simulink model "sensorless"  (R2018b)
settings: Solver=ode45  StartTime=0.0  StopTime=0.5  RelTol=1e-3  EnableMultiTasking=on
InitFcn:
  | tpwm=0.0001;
  | K=0.0604;
  | L1=0.00248;
  | L2=-1.239e-7*40;
  | Td=0;
  | kr=50;
  | wc=5;
  | speedref=10;
  | L1=0.00248;
  | L2=-1.239e-7*200;
libraries: dspsigops x72, powerlib x31, powerlib_meascontrol x24, simulink x8, powerlib_extras x5
(part 1 of 2)
settings Model: SimulationMode=accelerator  Creator=Administrator  LastModifiedBy=chenhao
settings DataIOCC: LimitDataPoints=on  SaveFormat=Array
settings OptimizationCC: EfficientMapNaN2IntZero=off  LifeSpan=inf
settings DebuggingCC: UnderspecifiedInitializationDetection=Classic  MergeDetectMultiDrivingBlocksExec=none  SolverPrmCheckMsg=warning  AllowSymbolicDim=off  SFUnexpectedBacktrackingDiag=warning  SFNoUnconditionalDefaultTransitionDiag=warning  SFExecutionAtInitializationDiag=none
settings HardwareCC: ProdBitPerPointer=32  ProdBitPerSizeT=32  ProdBitPerPtrDiffT=32  ProdLargestAtomicFloat=None  ProdIntDivRoundTo=Undefined  ProdEndianess=Unspecified  ProdWordSize=32  ProdHWDeviceType=32-bit Generic  TargetBitPerPointer=64  TargetBitPerSizeT=64  TargetBitPerPtrDiffT=64  TargetLongLongMode=on  TargetIntDivRoundTo=Zero  TargetEndianess=LittleEndian  TargetWordSize=64  TargetHWDeviceType=MATLAB Host  ProdEqTarget=off
settings ModelReferenceCC: PropagateSignalLabelsOutOfModel=off
settings SFSimCC: SimUseLocalCustomCode=off
settings RTWCC: RTWUseLocalCustomCode=off
settings CodeAppCC: MaxIdLength=128  StateflowObjectComments=on
settings GRTTargetCC: TargetLangStandard=C89/C90 (ANSI)  CombineOutputUpdateFcns=off  GRTInterface=on
settings ConfigComp: CovMetricSettings=dw  CovHtmlReporting=on  CovSaveCumulativeToWorkspaceVar=on  CovSaveSingleToWorkspaceVar=on  CovExternalEMLEnable=off
settings SimscapeCC: SimscapeNormalizeSystem=off

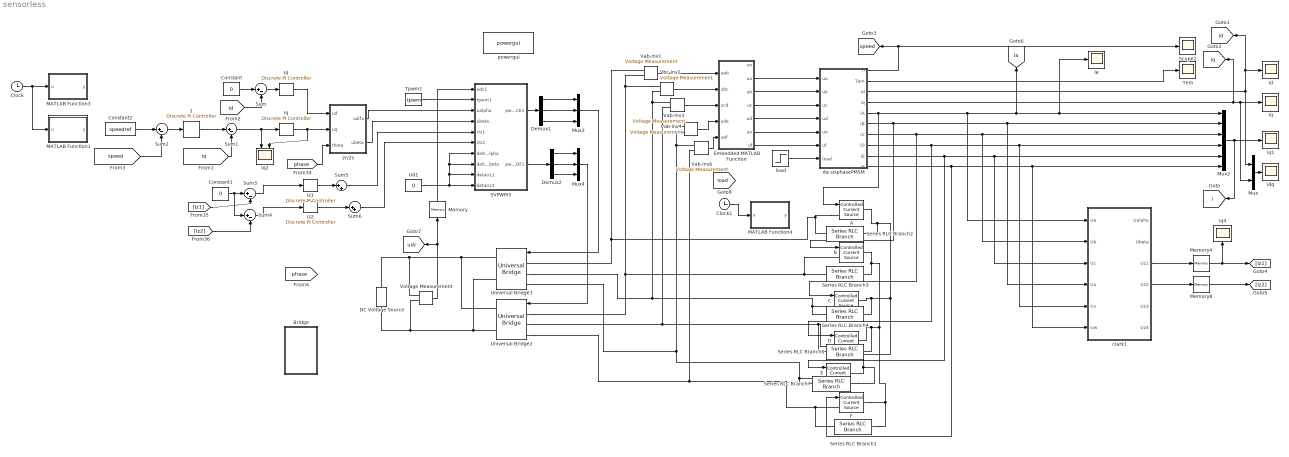
== system sensorless ==
  "    1" : powerlib_extras/Discrete  Control Blocks/Discrete PI Controller  Kp=1  Ki=80  Par_Limits=[50 -50]  Init=0  Ts=tpwm
  " Id" : powerlib_extras/Discrete  Control Blocks/Discrete PI Controller  Kp=3  Ki=120  Par_Limits=[300 -300]  Init=0  Ts=tpwm
  " Iq" : powerlib_extras/Discrete  Control Blocks/Discrete PI Controller  Kp=3  Ki=120  Par_Limits=[300 -300]  Init=0  Ts=tpwm
  " iz1" : powerlib_extras/Discrete  Control Blocks/Discrete PI Controller  Kp=10  Ki=100  Par_Limits=[300 -300]  Init=0  Ts=tpwm
  " iz2" : powerlib_extras/Discrete  Control Blocks/Discrete PI Controller  Kp=10  Ki=100  Par_Limits=[300 -300]  Init=0  Ts=tpwm
  2r/2s : Subsystem
  A : powerlib/Electrical Sources/Controlled Current Source  Initialize=on  Source_Type=AC  Amplitude=0  Phase=0  Frequency=0  Measurements=None
  B : powerlib/Electrical Sources/Controlled Current Source  Initialize=on  Source_Type=AC  Amplitude=0  Phase=0  Frequency=0  Measurements=None
  Bridge : Subsystem
  C : powerlib/Electrical Sources/Controlled Current Source  Initialize=on  Source_Type=AC  Amplitude=0  Phase=0  Frequency=0  Measurements=None
  Clock : Clock
  Clock1 : Clock
  Constant : Constant  Value=0
  Constant1 : Constant  Value=0
  Constant2 : Constant  Value=speedref
  D : powerlib/Electrical Sources/Controlled Current Source  Initialize=on  Source_Type=AC  Amplitude=0  Phase=0  Frequency=0  Measurements=None
  DC Voltage Source : powerlib/Electrical Sources/DC Voltage Source  Amplitude=100  Measurements=Voltage
  Demux1 : Demux  Outputs=3
  Demux2 : Demux  Outputs=3
  E : powerlib/Electrical Sources/Controlled Current Source  Initialize=on  Source_Type=AC  Amplitude=0  Phase=0  Frequency=0  Measurements=None
  Embedded MATLAB Function : MATLAB Function  TreatAsAtomicUnit=on
  F : powerlib/Electrical Sources/Controlled Current Source  Initialize=on  Source_Type=AC  Amplitude=0  Phase=0  Frequency=0  Measurements=None
  Ia : Scope
  MATLAB Function1 : MATLAB Function  TreatAsAtomicUnit=on
  MATLAB Function3 : MATLAB Function  TreatAsAtomicUnit=on
  MATLAB Function4 : MATLAB Function  TreatAsAtomicUnit=on
  Memory : Memory
  Memory4 : Memory
  Memory8 : Memory
  Mux : Mux  Inputs=2
  Mux2 : Mux  Inputs=6
  Mux3 : Mux  Inputs=3
  Mux4 : Mux  Inputs=3
  SVPWM3 : Subsystem
  Scope2 : Scope
  Series RLC Branch{1..4,6..7} (6 alike) : powerlib/Elements/Series RLC Branch  LConnTagsString=__new0  RConnTagsString=__new0  BranchType=R  Resistance=10e10  Inductance=10e-7  SetiL0=off  InitialCurrent=0  Capacitance=1e-6  Setx0=off  InitialVoltage=0  Measurements=None
  Sum{,1..4} (5 alike) : Sum  Inputs=|+-
  Sum5 : Sum  Inputs=|++
  Sum6 : Sum  Inputs=|++
  Tem : Scope
  Tpwm1 : Constant  Value=tpwm
  Ud1 : Constant  Value=0
  Universal Bridge1 : powerlib/Power Electronics/Universal Bridge  Arms=3  SnubberResistance=1e5  SnubberCapacitance=inf  Device=IGBT / Diodes  Ron=1e-3  Lon=0  ForwardVoltages="[  0  0  ]"  ForwardVoltage=0  GTOparameters=[ 10e-6 , 20e-6 ]  IGBTparameters=[ 0 , 0 ]  Measurements=None  Measurements_2=None  converterType=Rectifier
  Universal Bridge2 : powerlib/Power Electronics/Universal Bridge  Arms=3  SnubberResistance=1e5  SnubberCapacitance=inf  Device=IGBT / Diodes  Ron=1e-3  Lon=0  ForwardVoltages="[  0  0  ]"  ForwardVoltage=0  GTOparameters=[ 10e-6 , 20e-6 ]  IGBTparameters=[ 0 , 0 ]  Measurements=None  Measurements_2=None  converterType=Rectifier
  Vab-inv{1,3..4,6} (4 alike) : powerlib/Measurements/Voltage Measurement  Tag=PoWeRsYsTeMmEaSuReMeNt  PhasorSimulation=off  OutputType=Magnitude  PSBequivalent=0
  Vbc-inv2 : powerlib/Measurements/Voltage Measurement  Tag=PoWeRsYsTeMmEaSuReMeNt  PhasorSimulation=off  OutputType=Magnitude  PSBequivalent=0
  Voltage Measurement : powerlib/Measurements/Voltage Measurement  PhasorSimulation=off  OutputType=Complex  PSBequivalent=0
  clark1 : MATLAB Function  TreatAsAtomicUnit=on
  dq-sixphasePMSM : Subsystem  mask{R=0.099, Ld=2.463342136542000e-03, Lq=2.473254136542000e-03, Lf=1.520747e-3, psi=0.0592, p=5, J=0.00174}
      mask prompts: R "Resistance (Om)"; Ld "d-inductance (H)"; Lq "q-inductance (H)"; Lf "Leak inductance (H)"; psi "flux (Wb)"; p "pole pairs"; J "inertia (kg*m^2)"
  id : Scope
  idq : Scope
  iq : Scope
  iq1 : Scope
  iq2 : Scope  NumInputPorts=2
  iq4 : Scope
  load : Step  Time=0.1  After=5  SampleTime=0
  powergui : powerlib/powergui  Priority=1  SimulationMode=Discrete  SampleTime=5e-7  frequency=60  Iterations=50  frequencyindice=0  Pbase=100e6  ErrMax=1e-4  UnitsV=kV  UnitsW=MW  buscounter=0  FunctionMessages=off  echomessages=off  EnableUseOfTLC=off  CurrentSourceSwitches=off  DisableSnubberDevices=off  DisableRonSwitches=off  DisableVfSwitches=off  DisplayEquations=off  SolverType=Tustin  Interpol=off  ExternalGateDelay=off  methode=off  Ts=0  x0status=blocks  SPID=off  SwTol=0  HookPort=off  RestoreLinks=warning  ResistiveCurrentMeasurement=off  Frange=[0:2:500]  Ylog=off  Xlog=on  ShowGrid=off  save=off  variable=ZData  structure=Ia  ZoomFFT=on  StartTime=0.1  cycles=2  DisplayStyle=1  fundamental=2.5  FreqAxis=on  MaxFrequency=30  frequencyindicesteady=1  RmsSteady=1  display=off
  tag scope: Ia=global, i=global, id=global, iq=global, load=global, speed=global, udc=global
  wires:
  Vab-inv1/1 -> Embedded MATLAB Function/1(uab)
  Vbc-inv2/1 -> Embedded MATLAB Function/2(ubc)
  Vab-inv3/1 -> Embedded MATLAB Function/3(ucd)
  Vab-inv4/1 -> Embedded MATLAB Function/4(ude)
  Vab-inv6/1 -> Embedded MATLAB Function/5(uef)
  Embedded MATLAB Function/2(ua) -> dq-sixphasePMSM/1(ua)
  Embedded MATLAB Function/3(ub) -> dq-sixphasePMSM/2(ub)
  Embedded MATLAB Function/4(uc) -> dq-sixphasePMSM/3(uc)
  Embedded MATLAB Function/5(ud) -> dq-sixphasePMSM/4(ud)
  Embedded MATLAB Function/6(ue) -> dq-sixphasePMSM/5(ue)
  Embedded MATLAB Function/7(uf) -> dq-sixphasePMSM/6(uf)
  Mux/1 -> idq/1
  Sum1/1 -> iq2/1, " Iq"/1
  Constant/1 -> Sum/1
  Sum2/1 -> "    1"/1
  [phase] -> 2r/2s/3(theta)
  Mux3/1 -> Universal Bridge1/1
  Demux1/2 -> Mux3/2
  Mux4/1 -> Universal Bridge2/1
  Mux2/1 -> iq1/1, [i]
  "    1"/1 -> Sum1/1
  Sum/1 -> " Id"/1
  " Id"/1 -> 2r/2s/1(ud)
  " Iq"/1 -> iq2/2, 2r/2s/2(uq)
  Demux2/2 -> Mux4/2
  Demux2/1 -> Mux4/1
  Demux1/3 -> Mux3/3
  Demux2/3 -> Mux4/3
  Voltage Measurement/1 -> [udc], Memory/1
  SVPWM3/1(pwm_ACE1) -> Demux1/1
  SVPWM3/2(pwm_BDF1) -> Demux2/1
  dq-sixphasePMSM/1(n) -> Scope2/1, [speed]
  dq-sixphasePMSM/2(Tem) -> Tem/1
  dq-sixphasePMSM/3(id) -> [id], id/1, Mux/1
  dq-sixphasePMSM/4(iq) -> [iq], Mux/2, iq/1
  dq-sixphasePMSM/5(iA) -> A/1, clark1/1(Ua), [Ia], Ia/1, Mux2/1
  dq-sixphasePMSM/6(iB) -> B/1, clark1/4(Uu), Mux2/2
  dq-sixphasePMSM/7(iC) -> C/1, clark1/2(Ub), Mux2/3
  dq-sixphasePMSM/8(iD) -> D/1, clark1/5(Uv), Mux2/4
  dq-sixphasePMSM/10(iF) -> F/1, clark1/6(Uw), Mux2/6
  dq-sixphasePMSM/9(iE) -> E/1, clark1/3(Uc), Mux2/5
  [id] -> Sum/2
  [iq] -> Sum1/2
  Tpwm1/1 -> SVPWM3/2(tpwm1)
  Memory/1 -> SVPWM3/1(udc1)
  2r/2s/1(ualfa) -> SVPWM3/3(ualpha)
  2r/2s/2(ubeta) -> SVPWM3/4(ubeta)
  Constant1/1 -> Sum4/1, Sum3/1
  Sum3/1 -> " iz1"/1
  Sum4/1 -> " iz2"/1
  Ud1/1 -> SVPWM3/9(detaUz1), SVPWM3/8(deltaUbeta), SVPWM3/7(deltaUalpha), SVPWM3/10(detaUz2)
  " iz1"/1 -> Sum5/1
  " iz2"/1 -> Sum6/1
  clark1/3(Uz1) -> Memory4/1
  clark1/4(Uz2) -> Memory8/1
  Memory4/1 -> [Iz1], iq4/1
  Memory8/1 -> [Iz2]
  [Iz1] -> Sum3/2
  [Iz2] -> Sum4/2
  Demux1/1 -> Mux3/1
  Clock/1 -> MATLAB Function1/1(u), MATLAB Function3/1(u)
  Clock1/1 -> MATLAB Function4/1(u)
  [speed] -> Sum2/2
  Sum5/1 -> SVPWM3/5(Uz1)
  Sum6/1 -> SVPWM3/6(Uz2)
  load/1 -> dq-sixphasePMSM/7(load)
  Constant2/1 -> Sum2/1
  connections:
  A/LConn1 -- Series RLC Branch2/LConn1 -- Universal Bridge1/LConn1 -- Vab-inv1/LConn1
  Vbc-inv2/LConn1 -- Universal Bridge2/LConn1 -- Series RLC Branch3/LConn1 -- B/LConn1 -- Vab-inv1/LConn2
  C/LConn1 -- Universal Bridge1/LConn2 -- Vbc-inv2/LConn2 -- Vab-inv3/LConn1 -- Series RLC Branch4/LConn1
  Vab-inv4/LConn1 -- Vab-inv3/LConn2 -- Series RLC Branch6/LConn1 -- D/LConn1 -- Universal Bridge2/LConn2
  E/LConn1 -- Universal Bridge1/LConn3 -- Vab-inv4/LConn2 -- Vab-inv6/LConn1 -- Series RLC Branch7/LConn1
  Series RLC Branch1/LConn1 -- F/LConn1 -- Universal Bridge2/LConn3 -- Vab-inv6/LConn2
  Series RLC Branch1/RConn1 -- F/RConn1 -- Series RLC Branch3/RConn1 -- B/RConn1 -- Series RLC Branch6/RConn1 -- D/RConn1
  Series RLC Branch7/RConn1 -- E/RConn1 -- Series RLC Branch2/RConn1 -- A/RConn1 -- Series RLC Branch4/RConn1 -- C/RConn1
  Universal Bridge2/RConn2 -- DC Voltage Source/LConn1 -- Voltage Measurement/LConn2 -- Universal Bridge1/RConn2
  Universal Bridge2/RConn1 -- Universal Bridge1/RConn1 -- DC Voltage Source/RConn1 -- Voltage Measurement/LConn1

== system sensorless/2r//2s ==
  ud : Inport
  uq : Inport  Port=2
  theta : Inport  Port=3
  Fcn : Fcn  Expr=u(1)*cos(u(3))-u(2)*sin(u(3))
  Fcn1 : Fcn  Expr=u(1)*sin(u(3))+u(2)*cos(u(3))
  Mux1 : Mux  Inputs=3
  ualfa : Outport
  ubeta : Outport  Port=2
  wires:
  theta/1 -> Mux1/3
  uq/1 -> Mux1/2
  ud/1 -> Mux1/1
  Fcn1/1 -> ubeta/1
  Fcn/1 -> ualfa/1
  Mux1/1 -> Fcn1/1, Fcn/1

== system sensorless/Bridge ==
  100uF : powerlib/Elements/Series RLC Branch  LConnTagsString=__new0  RConnTagsString=__new0  BranchType=C  Resistance=1  Inductance=1e-3  SetiL0=off  InitialCurrent=0  Capacitance=1000e-6  Setx0=on  InitialVoltage=500  Measurements=None
  Diode{,1..5} (6 alike) : powerlib/Power Electronics/Diode  Ron=0.001  Lon=0  Vf=0.8  IC=0  UseSnubber=off  Rs=500  Cs=250e-9  Measurements=on
  Three-Phase Source1 : powerlib/Electrical Sources/Three-Phase Source  InternalConnection=Yg  VoltagePhases=off  Voltage=380  PhaseAngle=0  Voltage_phases=[25e3 25e3 25e3]/sqrt(3)  PhaseAngles_phases=[0 -120 +120]  Frequency=50  NonIdealSource=on  SpecifyImpedance=off  Resistance=1  Inductance=0.0000075  ShortCircuitLevel=100e6  BaseVoltage=380  XRratio=7  BusType=swing  Pref=0  Qref=0  Prefabc=[10e3, 10e3, 10e3]  Qrefabc=[0, 0, 0]  Qmin=-inf  Qmax=inf
  filter : powerlib/Elements/Series RLC Branch  LConnTagsString=__new0  RConnTagsString=__new0  BranchType=L  Resistance=1  Inductance=1e-6  SetiL0=off  InitialCurrent=0  Capacitance=1e-6  Setx0=off  InitialVoltage=0  Measurements=None
  +Vdc : PMIOPort  Tag=PMCPort  Side=Left
  -Vdc : PMIOPort  Tag=PMCPort  Port=2  Side=Right
  connections:
  filter/LConn1 -- Diode1/RConn1 -- Diode/RConn1 -- Diode4/RConn1
  Diode3/LConn1 -- Diode5/LConn1 -- Diode2/LConn1 -- 100uF/RConn1 -- -Vdc/RConn1
  Three-Phase Source1/RConn1 -- Diode2/RConn1 -- Diode/LConn1
  Diode3/RConn1 -- Three-Phase Source1/RConn3 -- Diode4/LConn1
  Three-Phase Source1/RConn2 -- Diode5/RConn1 -- Diode1/LConn1
  100uF/LConn1 -- +Vdc/RConn1 -- filter/RConn1

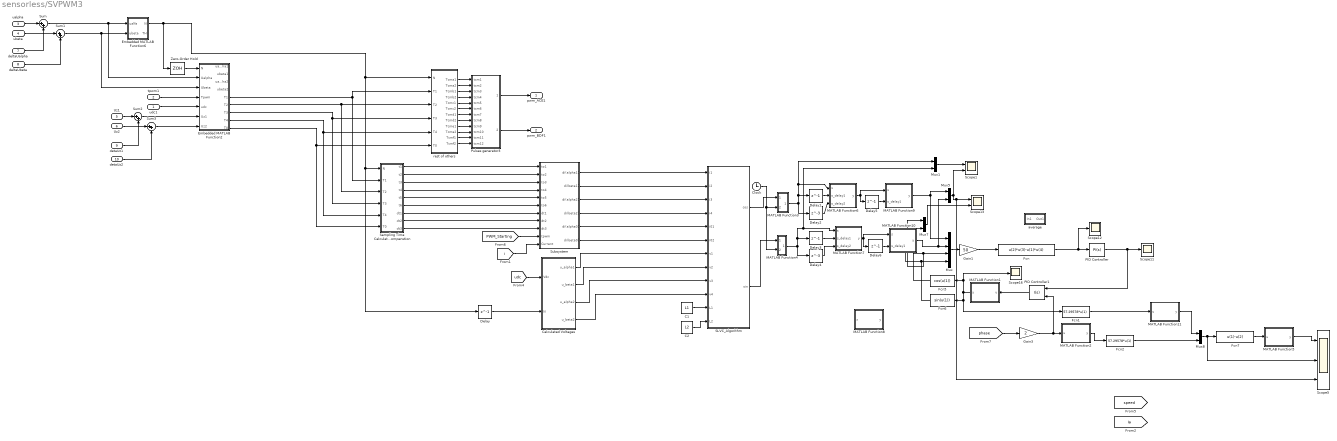
== system sensorless/SVPWM3 ==
  udc1 : Inport
  tpwm1 : Inport  Port=2
  ualpha : Inport  Port=3
  ubeta : Inport  Port=4
  Uz1 : Inport  Port=5
  Uz2 : Inport  Port=6
  deltaUalpha : Inport  Port=7
  deltaUbeta : Inport  Port=8
  detaUz1 : Inport  Port=9
  detaUz2 : Inport  Port=10
  C1 : Constant  Value=L1
  C2 : Constant  Value=L2
  "Calculated Voltages " : Subsystem
  Clock : Clock
  Delay{,1,3,5..6} (5 alike) : Delay  DelayLength=1  InitialCondition=0  SampleTime=1e-4
  Delay2 : Delay  DelayLength=3  InitialCondition=0  SampleTime=1e-4
  Delay4 : Delay  DelayLength=3  InitialCondition=0  SampleTime=1e-4
  Embedded MATLAB Function2 : MATLAB Function  TreatAsAtomicUnit=on
  Embedded MATLAB Function6 : MATLAB Function  TreatAsAtomicUnit=on
  Fcn : Fcn  Expr=u(2)*u(3)-u(1)*u(4)
  Fcn1 : Fcn  Expr=57.29578*u(1)
  Fcn2 : Fcn  Expr=57.29578*u(1)
  Fcn5 : Fcn  Expr=cos(u(1))
  Fcn6 : Fcn  Expr=sin(u(1))
  Fcn7 : Fcn  Expr=u(1)-u(2)
  Gain1 : Gain  Gain=50
  Gain3 : Gain  Gain=2
  MATLAB Function1 : MATLAB Function  TreatAsAtomicUnit=on
  MATLAB Function10 : MATLAB Function  TreatAsAtomicUnit=on
  MATLAB Function11 : MATLAB Function  TreatAsAtomicUnit=on
  MATLAB Function2 : MATLAB Function  TreatAsAtomicUnit=on
  MATLAB Function3 : MATLAB Function  TreatAsAtomicUnit=on
  MATLAB Function4 : MATLAB Function  TreatAsAtomicUnit=on
  MATLAB Function5 : MATLAB Function  TreatAsAtomicUnit=on
  MATLAB Function6 : MATLAB Function  TreatAsAtomicUnit=on
  MATLAB Function7 : MATLAB Function  TreatAsAtomicUnit=on
  MATLAB Function8 : MATLAB Function  TreatAsAtomicUnit=on
  MATLAB Function9 : MATLAB Function  TreatAsAtomicUnit=on
  Mux : Mux
  Mux{1,5,7..8} (4 alike) : Mux  Inputs=2
  PID Controller : simulink/Continuous/PID Controller  Controller=PI  Form=Parallel  TimeDomain=Continuous-time  SampleTime=-1  IntegratorMethod=Forward Euler  FilterMethod=Forward Euler  ControllerParametersSource=internal  P=1  I=100  D=0  UseFilter=on  N=100  TunerSelectOption=Transfer Function Based (PID Tuner App)  InitialConditionSource=internal  InitialConditionForIntegrator=1  InitialConditionForFilter=0  DifferentiatorICPrevScaledInput=0  ExternalReset=none  TrackingMode=off  Kt=1  LimitOutput=off  UpperSaturationLimit=200  LowerSaturationLimit=-200  LinearizeAsGain=on  AntiWindupMode=none  Kb=1  POutMin=[]  POutMax=[]  IOutMin=[]  IOutMax=[]  DOutMin=[]  DOutMax=[]  NOutMin=[]  NOutMax=[]  SumOutMin=[]  SumOutMax=[]  SaturationOutMin=[]  SaturationOutMax=[]  PParamMin=[]  PParamMax=[]  IParamMin=[]  IParamMax=[]  DParamMin=[]  DParamMax=[]  NParamMin=[]  NParamMax=[]  KbParamMin=[]  KbParamMax=[]  KtParamMin=[]  KtParamMax=[]  KbOutMin=[]  KbOutMax=[]  KtOutMin=[]  KtOutMax=[]  IntegratorOutMin=[]  IntegratorOutMax=[]  FilterOutMin=[]  FilterOutMax=[]  SumI1OutMin=[]  SumI1OutMax=[]  SumI2OutMin=[]  SumI2OutMax=[]  SumI3OutMin=[]  SumI3OutMax=[]  SumI4OutMin=[]  SumI4OutMax=[]  SumDOutMin=[]  SumDOutMax=[]  DifferentiatorOutMin=[]  DifferentiatorOutMax=[]  FilterDiffOutCoefMin=[]  FilterDiffOutCoefMax=[]  ReciprocalOutMin=[]  ReciprocalOutMax=[]  SumDenOutMin=[]  SumDenOutMax=[]  SumNumOutMin=[]  SumNumOutMax=[]  DivideOutMin=[]  DivideOutMax=[]  IntegratorContinuousStateAttributes=''  IntegratorStateMustResolveToSignalObject=off  IntegratorRTWStateStorageClass=Auto  FilterContinuousStateAttributes=''  FilterStateMustResolveToSignalObject=off  FilterRTWStateStorageClass=Auto  ParallelPVariant=InternalParameters  IdealPVariant=Disabled  IVariant=InternalParameters  DVariant=Disabled  IntegratorVariant=Continuous  SatVariant=Disabled  AWVariant=Passthrough  PCopyVariant=Disabled  TRVariant=Disabled  FdbkBlocksVariant=Forward  IdealPFdbkVariant=Disabled  SatFdbkVariant=Disabled  DerivativeFilterVariant=Disabled  NVariant=Disabled  NCopyVariant=Disabled_SignalSpec  FilterICVariant=Disabled  IntegratorICVariant=InternalICs  ExternalResetVariant=Disabled  TRSumVariant=Passthrough  SumFdbkVariant=Disabled  SumVariant=Sum_PI
  PID Controller1 : simulink/Continuous/PID Controller  Controller=I  Form=Parallel  TimeDomain=Continuous-time  SampleTime=-1  IntegratorMethod=Forward Euler  FilterMethod=Forward Euler  ControllerParametersSource=internal  P=1  I=1  D=0  UseFilter=on  N=100  TunerSelectOption=Transfer Function Based (PID Tuner App)  InitialConditionSource=external  InitialConditionForIntegrator=0  InitialConditionForFilter=0  DifferentiatorICPrevScaledInput=0  ExternalReset=none  TrackingMode=off  Kt=1  LimitOutput=off  UpperSaturationLimit=inf  LowerSaturationLimit=-inf  LinearizeAsGain=on  AntiWindupMode=none  Kb=1  POutMin=[]  POutMax=[]  IOutMin=[]  IOutMax=[]  DOutMin=[]  DOutMax=[]  NOutMin=[]  NOutMax=[]  SumOutMin=[]  SumOutMax=[]  SaturationOutMin=[]  SaturationOutMax=[]  PParamMin=[]  PParamMax=[]  IParamMin=[]  IParamMax=[]  DParamMin=[]  DParamMax=[]  NParamMin=[]  NParamMax=[]  KbParamMin=[]  KbParamMax=[]  KtParamMin=[]  KtParamMax=[]  KbOutMin=[]  KbOutMax=[]  KtOutMin=[]  KtOutMax=[]  IntegratorOutMin=[]  IntegratorOutMax=[]  FilterOutMin=[]  FilterOutMax=[]  SumI1OutMin=[]  SumI1OutMax=[]  SumI2OutMin=[]  SumI2OutMax=[]  SumI3OutMin=[]  SumI3OutMax=[]  SumI4OutMin=[]  SumI4OutMax=[]  SumDOutMin=[]  SumDOutMax=[]  DifferentiatorOutMin=[]  DifferentiatorOutMax=[]  FilterDiffOutCoefMin=[]  FilterDiffOutCoefMax=[]  ReciprocalOutMin=[]  ReciprocalOutMax=[]  SumDenOutMin=[]  SumDenOutMax=[]  SumNumOutMin=[]  SumNumOutMax=[]  DivideOutMin=[]  DivideOutMax=[]  IntegratorContinuousStateAttributes=''  IntegratorStateMustResolveToSignalObject=off  IntegratorRTWStateStorageClass=Auto  FilterContinuousStateAttributes=''  FilterStateMustResolveToSignalObject=off  FilterRTWStateStorageClass=Auto  ParallelPVariant=Disabled  IdealPVariant=Disabled  IVariant=InternalParameters  DVariant=Disabled  IntegratorVariant=Continuous  SatVariant=Disabled  AWVariant=Passthrough  PCopyVariant=Disabled  TRVariant=Disabled  FdbkBlocksVariant=Forward  IdealPFdbkVariant=Disabled  SatFdbkVariant=Disabled  DerivativeFilterVariant=Disabled  NVariant=Disabled  NCopyVariant=Disabled_SignalSpec  FilterICVariant=Disabled  IntegratorICVariant=ExternalICs  ExternalResetVariant=Disabled  TRSumVariant=Passthrough  SumFdbkVariant=Disabled  SumVariant=Passthrough_I
  Pulses generator3 : Subsystem
  SLVC_Algorithm : MATLAB Function  TreatAsAtomicUnit=on
  "Sampling Time Calculatuons & delayed compenstion " : Subsystem
  Scope1 : Scope  NumInputPorts=2
  Scope11 : Scope
  Scope12 : Scope
  Scope13 : Scope  NumInputPorts=2
  Scope16 : Scope
  Scope5 : Scope  NumInputPorts=3
  Subsystem : Subsystem
  Sum{,1..3} (4 alike) : Sum  Inputs=|++
  Zero-Order Hold : ZeroOrderHold  SampleTime=1e-4
  average : Subsystem
  rest of others : MATLAB Function  TreatAsAtomicUnit=on
  pwm_ACE1 : Outport
  pwm_BDF1 : Outport  Port=2
  wires:
  udc1/1 -> Embedded MATLAB Function2/5(udc)
  Embedded MATLAB Function2/8(T4) -> rest of others/5(T4), "Sampling Time Calculatuons & delayed compenstion "/5(T4)
  Embedded MATLAB Function2/5(T1) -> rest of others/2(T1), "Sampling Time Calculatuons & delayed compenstion "/2(T1)
  Pulses generator3/1(pwm_ACE) -> pwm_ACE1/1
  Pulses generator3/2(pwm_BDF) -> pwm_BDF1/1
  rest of others/12(Tcmf2) -> Pulses generator3/12(tcm12)
  rest of others/11(Tcmf1) -> Pulses generator3/11(tcm11)
  rest of others/10(Tcme2) -> Pulses generator3/10(tcm10)
  rest of others/9(Tcme1) -> Pulses generator3/9(tcm9)
  rest of others/8(Tcmd2) -> Pulses generator3/8(tcm8)
  rest of others/7(Tcmd1) -> Pulses generator3/7(tcm7)
  rest of others/6(Tcmc2) -> Pulses generator3/6(tcm6)
  rest of others/5(Tcmc1) -> Pulses generator3/5(tcm5)
  rest of others/4(Tcmb2) -> Pulses generator3/4(tcm4)
  rest of others/3(Tcmb1) -> Pulses generator3/3(tcm3)
  rest of others/2(Tcma2) -> Pulses generator3/2(tcm2)
  rest of others/1(Tcma1) -> Pulses generator3/1(tcm1)
  Embedded MATLAB Function2/6(T2) -> "Sampling Time Calculatuons & delayed compenstion "/3(T2), rest of others/3(T2)
  tpwm1/1 -> Embedded MATLAB Function2/4(Tpwm)
  Embedded MATLAB Function2/9(T0) -> rest of others/6(T0), "Sampling Time Calculatuons & delayed compenstion "/6(T0)
  ualpha/1 -> Sum/1
  deltaUalpha/1 -> Sum/2
  Sum/1 -> Embedded MATLAB Function2/2(Ualpha), Embedded MATLAB Function6/1(ualfa)
  ubeta/1 -> Sum1/1
  Sum1/1 -> Embedded MATLAB Function2/3(Ubeta), Embedded MATLAB Function6/2(ubeta)
  deltaUbeta/1 -> Sum1/2
  Uz1/1 -> Sum2/1
  Sum2/1 -> Embedded MATLAB Function2/6(Uz1)
  detaUz1/1 -> Sum2/2
  Uz2/1 -> Sum3/1
  Sum3/1 -> Embedded MATLAB Function2/7(Uz2)
  detaUz2/1 -> Sum3/2
  Embedded MATLAB Function2/7(T3) -> "Sampling Time Calculatuons & delayed compenstion "/4(T3), rest of others/4(T3)
  "Sampling Time Calculatuons & delayed compenstion "/1(t1) -> Subsystem/1(to1)
  "Sampling Time Calculatuons & delayed compenstion "/2(t2) -> Subsystem/2(to2)
  "Sampling Time Calculatuons & delayed compenstion "/3(t3) -> Subsystem/3(to3)
  "Sampling Time Calculatuons & delayed compenstion "/4(t4) -> Subsystem/4(to4)
  "Sampling Time Calculatuons & delayed compenstion "/5(t5) -> Subsystem/5(to5)
  "Sampling Time Calculatuons & delayed compenstion "/6(t6) -> Subsystem/6(to6)
  [PWM_Starting] -> Subsystem/10(tpwm)
  [i] -> Subsystem/11(Current)
  [udc] -> "Calculated Voltages "/1(Vdc)
  "Calculated Voltages "/1(u_alpha1) -> SLVC_Algorithm/7(v1)
  "Calculated Voltages "/2(u_beta1) -> SLVC_Algorithm/8(v2)
  "Calculated Voltages "/3(u_alpha2) -> SLVC_Algorithm/9(v3)
  "Calculated Voltages "/4(u_beta2) -> SLVC_Algorithm/10(v4)
  C1/1 -> SLVC_Algorithm/11(L1)
  C2/1 -> SLVC_Algorithm/12(L2)
  Subsystem/3(di(alpha2)) -> SLVC_Algorithm/3(i3)
  Subsystem/2(di(beta1)) -> SLVC_Algorithm/2(i2)
  Subsystem/4(di(beta2)) -> SLVC_Algorithm/4(i4)
  Subsystem/5(di(alpha0)) -> SLVC_Algorithm/5(i01)
  Subsystem/1(di(alpha1)) -> SLVC_Algorithm/1(i1)
  Subsystem/6(di(beta0)) -> SLVC_Algorithm/6(i02)
  "Sampling Time Calculatuons & delayed compenstion "/7(dt1) -> Subsystem/7(dt1)
  "Sampling Time Calculatuons & delayed compenstion "/8(dt2) -> Subsystem/8(dt2)
  "Sampling Time Calculatuons & delayed compenstion "/9(dt3) -> Subsystem/9(dt3)
  Mux/1 -> Gain1/1
  PID Controller1/1 -> MATLAB Function1/1(u)
  Fcn6/1 -> Mux/4, Mux7/2
  PID Controller/1 -> PID Controller1/1, Scope11/1
  Gain1/1 -> Fcn/1
  [phase] -> Gain3/1
  MATLAB Function2/1(y) -> Fcn2/1
  Fcn7/1 -> MATLAB Function5/1(u)
  MATLAB Function5/1(y) -> Scope5/1
  Fcn/1 -> PID Controller/1, Scope12/1
  Gain3/1 -> PID Controller1/2, MATLAB Function2/1(u)
  Clock/1 -> MATLAB Function3/2(clock), MATLAB Function4/2(clock)
  SLVC_Algorithm/2(sin) -> MATLAB Function4/1(x)
  SLVC_Algorithm/1(cos) -> MATLAB Function3/1(x)
  Zero-Order Hold/1 -> Embedded MATLAB Function2/1(N)
  Embedded MATLAB Function6/1(N) -> rest of others/1(N), Delay/1, "Sampling Time Calculatuons & delayed compenstion "/1(N), Zero-Order Hold/1
  Delay/1 -> "Calculated Voltages "/2(N)
  Delay1/1 -> MATLAB Function6/2(s_delay1)
  Delay2/1 -> MATLAB Function6/3(s_delay2)
  Delay3/1 -> MATLAB Function7/2(s_delay1)
  Delay4/1 -> MATLAB Function7/3(s_delay2)
  MATLAB Function4/1(y) -> Delay3/1, Mux1/2, MATLAB Function7/1(s), Delay4/1
  MATLAB Function3/1(y) -> Mux1/1, MATLAB Function6/1(s), Delay1/1, Delay2/1
  Mux7/1 -> Scope13/2
  Fcn5/1 -> Mux7/1, Mux/3
  Mux1/1 -> Scope1/1
  Mux8/1 -> Scope5/2, Fcn7/1
  Mux5/1 -> Scope5/3, Scope13/1, Scope1/2
  MATLAB Function1/1(y) -> Fcn1/1, Fcn6/1, Fcn5/1, Scope16/1
  Fcn2/1 -> Mux8/2
  Delay5/1 -> MATLAB Function9/2(s_delay1)
  MATLAB Function9/1(y) -> Mux5/1, Mux/1
  MATLAB Function6/1(y) -> MATLAB Function9/1(s), Delay5/1
  Delay6/1 -> MATLAB Function10/2(s_delay1)
  MATLAB Function7/1(y) -> Delay6/1, MATLAB Function10/1(s)
  MATLAB Function10/1(y) -> Mux5/2, Mux/2
  MATLAB Function11/1(y) -> Mux8/1
  Fcn1/1 -> MATLAB Function11/1(u)

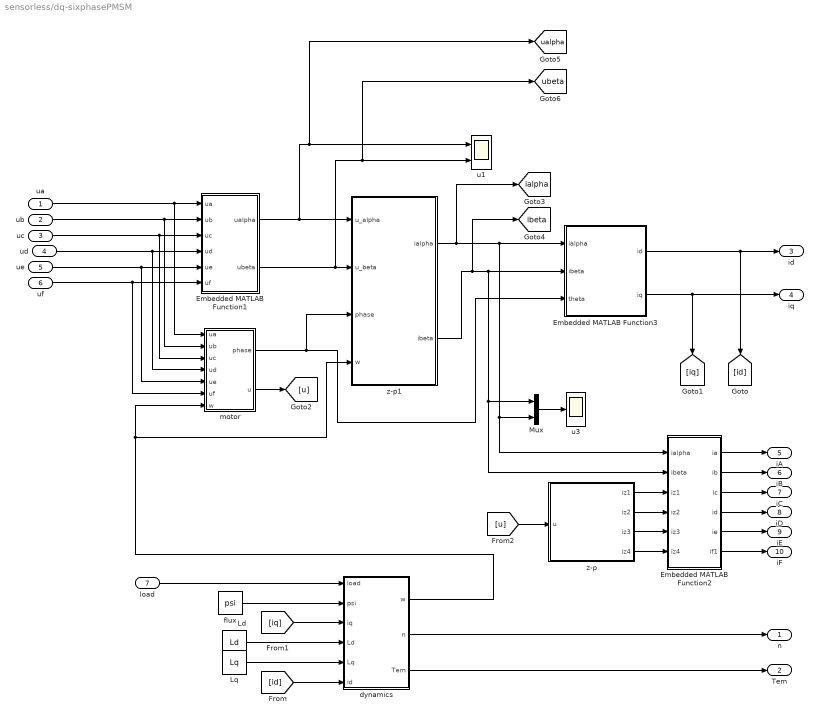
== system sensorless/dq-sixphasePMSM ==
  ua : Inport
  ub : Inport  Port=2
  uc : Inport  Port=3
  ud : Inport  Port=4
  ue : Inport  Port=5
  uf : Inport  Port=6
  load : Inport  Port=7
  Embedded MATLAB Function1 : MATLAB Function  TreatAsAtomicUnit=on
  Embedded MATLAB Function2 : MATLAB Function  TreatAsAtomicUnit=on
  Embedded MATLAB Function3 : MATLAB Function  TreatAsAtomicUnit=on
  Ld : Constant  Value=Ld
  Lq : Constant  Value=Lq
  Mux : Mux  Inputs=2
  dynamics : Subsystem
  flux : Constant  Value=psi
  motor : Subsystem
  u1 : Scope  NumInputPorts=2
  u3 : Scope
  z-p : Subsystem
  z-p1 : Subsystem
  n : Outport
  Tem : Outport  Port=2
  id : Outport  Port=3
  iq : Outport  Port=4
  iA : Outport  Port=5
  iB : Outport  Port=6
  iC : Outport  Port=7
  iD : Outport  Port=8
  iE : Outport  Port=9
  iF : Outport  Port=10
  tag scope: ialpha=global, ibeta=global, ualpha=global, ubeta=global
  wires:
  Embedded MATLAB Function2/3(ic) -> iC/1
  Embedded MATLAB Function2/5(ie) -> iE/1
  Embedded MATLAB Function2/4(id) -> iD/1
  Embedded MATLAB Function2/1(ia) -> iA/1
  Embedded MATLAB Function2/2(ib) -> iB/1
  Embedded MATLAB Function2/6(if1) -> iF/1
  ua/1 -> motor/1(ua), Embedded MATLAB Function1/1(ua)
  uc/1 -> motor/3(uc), Embedded MATLAB Function1/3(uc)
  ud/1 -> motor/4(ud), Embedded MATLAB Function1/4(ud)
  ue/1 -> motor/5(ue), Embedded MATLAB Function1/5(ue)
  uf/1 -> motor/6(uf), Embedded MATLAB Function1/6(uf)
  Ld/1 -> dynamics/4(Ld)
  Lq/1 -> dynamics/5(Lq)
  load/1 -> dynamics/1(load)
  flux/1 -> dynamics/2(psi)
  [id] -> dynamics/6(id)
  [iq] -> dynamics/3(iq)
  z-p/2(iz2) -> Embedded MATLAB Function2/4(iz2)
  z-p/1(iz1) -> Embedded MATLAB Function2/3(iz1)
  z-p/4(iz4) -> Embedded MATLAB Function2/6(iz4)
  z-p/3(iz3) -> Embedded MATLAB Function2/5(iz3)
  ub/1 -> motor/2(ub), Embedded MATLAB Function1/2(ub)
  [u] -> z-p/1(u)
  z-p1/1(ialpha) -> [ialpha], Mux/2, Embedded MATLAB Function2/1(ialpha), Embedded MATLAB Function3/1(ialpha)
  z-p1/2(ibeta) -> [ibeta], Mux/1, Embedded MATLAB Function2/2(ibeta), Embedded MATLAB Function3/2(ibeta)
  Embedded MATLAB Function3/1(id) -> [id], id/1
  Embedded MATLAB Function3/2(iq) -> iq/1, [iq]
  Mux/1 -> u3/1
  dynamics/1(w) -> z-p1/4(w), motor/7(w)
  dynamics/2(n) -> n/1
  dynamics/3(Tem) -> Tem/1
  motor/2(u) -> [u]
  motor/1(phase) -> Embedded MATLAB Function3/3(theta), z-p1/3(phase)
  Embedded MATLAB Function1/1(ualpha) -> [ualpha], u1/1, z-p1/1(u_alpha)
  Embedded MATLAB Function1/2(ubeta) -> [ubeta], u1/2, z-p1/2(u_beta)

== system sensorless/SVPWM3/Calculated Voltages  ==
  Vdc : Inport
  N : Inport  Port=2
  Scope : Scope
  V_alpha1 & V_beta1 : MATLAB Function  TreatAsAtomicUnit=on
  V_alpha2 & V_beta2 : MATLAB Function  TreatAsAtomicUnit=on
  u_alpha1 : Outport
  u_beta1 : Outport  Port=2
  u_alpha2 : Outport  Port=3
  u_beta2 : Outport  Port=4
  tag scope: v1=global, v2=global, v3=global, v4=global
  wires:
  N/1 -> V_alpha2 & V_beta2/2(N), V_alpha1 & V_beta1/2(N)
  Vdc/1 -> V_alpha2 & V_beta2/1(udc), V_alpha1 & V_beta1/1(udc)
  V_alpha1 & V_beta1/1(u_alpha1) -> [v1], u_alpha1/1
  V_alpha1 & V_beta1/2(u_beta1) -> [v2], u_beta1/1
  V_alpha2 & V_beta2/1(u_alpha2) -> [v3], u_alpha2/1
  V_alpha2 & V_beta2/2(u_beta2) -> Scope/1, [v4], u_beta2/1

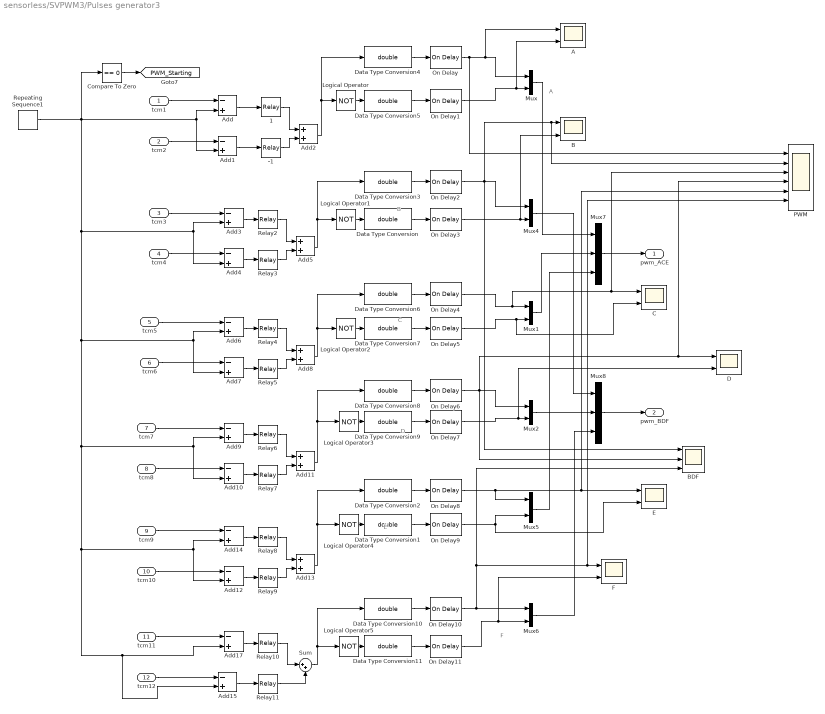
== system sensorless/SVPWM3/Pulses generator3 ==
  note: A
  note: B
  note: C
  note: D
  note: E
  note: F
  tcm1 : Inport
  tcm2 : Inport  Port=2
  tcm3 : Inport  Port=3
  tcm4 : Inport  Port=4
  tcm5 : Inport  Port=5
  tcm6 : Inport  Port=6
  tcm7 : Inport  Port=7
  tcm8 : Inport  Port=8
  tcm9 : Inport  Port=9
  tcm10 : Inport  Port=10
  tcm11 : Inport  Port=11
  tcm12 : Inport  Port=12
  -1 : Relay  OnOutputValue=-1
  1 : Relay
  A : Scope  NumInputPorts=2
  Add{,1,3..4,6..7,9..10,12,14..15,17} (12 alike) : Sum  Inputs=-+
  Add{2,5,8,11,13} (5 alike) : Sum
  B : Scope  NumInputPorts=2
  BDF : Scope  NumInputPorts=3
  C : Scope  NumInputPorts=2
  Compare To Zero : simulink/Logic and Bit Operations/Compare To Zero  relop===  OutDataTypeStr=boolean
  D : Scope  NumInputPorts=2
  Data Type Conversion{,1..11} (12 alike) : DataTypeConversion  OutDataTypeStr=double
  E : Scope  NumInputPorts=2
  F : Scope  NumInputPorts=2
  Logical Operator{,1..5} (6 alike) : Logic  Operator=NOT  AllPortsSameDT=off  OutDataTypeStr=boolean
  Mux{,1..2,4..6} (6 alike) : Mux  Inputs=2
  Mux7 : Mux  Inputs=3
  Mux8 : Mux  Inputs=3
  On Delay{,1..11} (12 alike) : powerlib_meascontrol/Logic/On Delay  DelayType=On delay  delay=Td  ic=0  Ts=0
      settings: SourceProductName=Simscape Power Systems
  PWM : Scope  NumInputPorts=6
  Relay{2,4,6,8,10} (5 alike) : Relay
  Relay{3,5,7,9,11} (5 alike) : Relay  OnOutputValue=-1
  Repeating Sequence1 : simulink/Sources/Repeating Sequence  rep_seq_t=[0 tpwm]  rep_seq_y=[0 tpwm]
  Sum : Sum  Inputs=|++
  pwm_ACE : Outport
  pwm_BDF : Outport  Port=2
  tag scope: PWM_Starting=global
  wires:
  On Delay11/1 -> F/2, Mux6/2
  Data Type Conversion11/1 -> On Delay11/1
  On Delay10/1 -> BDF/3, PWM/6, F/1, Mux6/1
  Data Type Conversion10/1 -> On Delay10/1
  On Delay9/1 -> E/2, Mux5/2
  Data Type Conversion1/1 -> On Delay9/1
  On Delay8/1 -> Mux5/1, PWM/5, E/1
  Data Type Conversion2/1 -> On Delay8/1
  On Delay7/1 -> D/2, Mux2/2
  Data Type Conversion9/1 -> On Delay7/1
  On Delay6/1 -> BDF/2, PWM/4, D/1, Mux2/1
  Data Type Conversion8/1 -> On Delay6/1
  On Delay5/1 -> C/2, Mux1/2
  Data Type Conversion7/1 -> On Delay5/1
  On Delay4/1 -> PWM/3, C/1, Mux1/1
  Data Type Conversion6/1 -> On Delay4/1
  On Delay2/1 -> BDF/1, PWM/2, B/1, Mux4/1
  On Delay3/1 -> B/2, Mux4/2
  Data Type Conversion/1 -> On Delay3/1
  Data Type Conversion3/1 -> On Delay2/1
  On Delay1/1 -> A/2, Mux/2
  Data Type Conversion5/1 -> On Delay1/1
  On Delay/1 -> A/1, Mux/1, PWM/1
  Data Type Conversion4/1 -> On Delay/1
  Logical Operator3/1 -> Data Type Conversion9/1
  Logical Operator2/1 -> Data Type Conversion7/1
  Logical Operator/1 -> Data Type Conversion5/1
  Logical Operator1/1 -> Data Type Conversion/1
  Logical Operator4/1 -> Data Type Conversion1/1
  Add5/1 -> Logical Operator1/1, Data Type Conversion3/1
  Add2/1 -> Logical Operator/1, Data Type Conversion4/1
  Mux8/1 -> pwm_BDF/1
  Mux7/1 -> pwm_ACE/1
  Mux/1 -> Mux7/1
  Sum/1 -> Logical Operator5/1, Data Type Conversion10/1
  Add13/1 -> Logical Operator4/1, Data Type Conversion2/1
  Add11/1 -> Logical Operator3/1, Data Type Conversion8/1
  Add8/1 -> Logical Operator2/1, Data Type Conversion6/1
  Logical Operator5/1 -> Data Type Conversion11/1
  tcm12/1 -> Add15/1
  Relay11/1 -> Sum/2
  Relay10/1 -> Sum/1
  Add17/1 -> Relay10/1
  tcm11/1 -> Add17/1
  tcm10/1 -> Add12/1
  Relay9/1 -> Add13/2
  Relay8/1 -> Add13/1
  Add12/1 -> Relay9/1
  Add14/1 -> Relay8/1
  tcm9/1 -> Add14/1
  tcm8/1 -> Add10/1
  Relay7/1 -> Add11/2
  Relay6/1 -> Add11/1
  Add10/1 -> Relay7/1
  Add9/1 -> Relay6/1
  tcm7/1 -> Add9/1
  tcm6/1 -> Add7/1
  Relay5/1 -> Add8/2
  Relay4/1 -> Add8/1
  Add7/1 -> Relay5/1
  Add6/1 -> Relay4/1
  tcm4/1 -> Add4/1
  Relay3/1 -> Add5/2
  Relay2/1 -> Add5/1
  Add4/1 -> Relay3/1
  Add3/1 -> Relay2/1
  tcm1/1 -> Add/1
  -1/1 -> Add2/2
  1/1 -> Add2/1
  Add1/1 -> -1/1
  Add/1 -> 1/1
  Repeating Sequence1/1 -> Compare To Zero/1, Add15/2, Add17/2, Add12/2, Add14/2, Add9/2, Add10/2, Add7/2, Add6/2, Add3/2, Add4/2, Add1/2, Add/2
  tcm2/1 -> Add1/1
  tcm3/1 -> Add3/1
  tcm5/1 -> Add6/1
  Mux4/1 -> Mux8/1
  Mux1/1 -> Mux7/2
  Mux2/1 -> Mux8/2
  Mux5/1 -> Mux7/3
  Mux6/1 -> Mux8/3
  Add15/1 -> Relay11/1
  Compare To Zero/1 -> [PWM_Starting]

== system sensorless/SVPWM3/Sampling Time Calculatuons & delayed compenstion  ==
  N : Inport
  T1 : Inport  Port=2
  T2 : Inport  Port=3
  T3 : Inport  Port=4
  T4 : Inport  Port=5
  T0 : Inport  Port=6
  Embedded MATLAB Function1 : MATLAB Function  TreatAsAtomicUnit=on
  Embedded MATLAB Function2 : MATLAB Function  TreatAsAtomicUnit=on
  Ialpha1 : Scope  NumInputPorts=3
  Ialpha4 : Scope  NumInputPorts=2
  Subsystem3 : Subsystem
  t{7..12} (6 alike) : powerlib_meascontrol/Logic/Edge Detector  model=Rising  ic=0  Ts=0
      settings: SourceProductName=Simscape Power Systems  SourceProductBaseCode=PS
  t1 : Outport
  t2 : Outport  Port=2
  t3 : Outport  Port=3
  t4 : Outport  Port=4
  t5 : Outport  Port=5
  t6 : Outport  Port=6
  dt1 : Outport  Port=7
  dt2 : Outport  Port=8
  dt3 : Outport  Port=9
  wires:
  N/1 -> Embedded MATLAB Function1/1(N)
  T1/1 -> Embedded MATLAB Function1/2(T1)
  T2/1 -> Embedded MATLAB Function1/3(T2)
  T3/1 -> Embedded MATLAB Function1/4(T3)
  T4/1 -> Embedded MATLAB Function1/5(T4)
  T0/1 -> Embedded MATLAB Function1/6(T0)
  Embedded MATLAB Function1/6(t6) -> Embedded MATLAB Function2/6(t6), Subsystem3/6(S6)
  Embedded MATLAB Function1/5(t5) -> Embedded MATLAB Function2/5(t5), Subsystem3/5(S5)
  Embedded MATLAB Function1/4(t4) -> Embedded MATLAB Function2/4(t4), Subsystem3/4(S4)
  Embedded MATLAB Function1/2(t2) -> Embedded MATLAB Function2/2(t2), Subsystem3/2(S2)
  Embedded MATLAB Function1/1(t1) -> Embedded MATLAB Function2/1(t1), Subsystem3/1(S1), Ialpha4/1
  Embedded MATLAB Function1/3(t3) -> Embedded MATLAB Function2/3(t3), Subsystem3/3(S3)
  Subsystem3/1(t1) -> Ialpha4/2, t7/1
  Subsystem3/2(t2) -> t8/1
  Subsystem3/3(t3) -> t9/1
  Subsystem3/4(t4) -> t10/1
  Subsystem3/5(t5) -> t11/1
  Subsystem3/6(t6) -> t12/1
  t7/1 -> t1/1
  t8/1 -> t2/1
  t9/1 -> t3/1
  t10/1 -> t4/1
  t11/1 -> t5/1
  t12/1 -> t6/1
  Embedded MATLAB Function2/2(dt2) -> Ialpha1/2, dt2/1
  Embedded MATLAB Function2/3(dt3) -> Ialpha1/3, dt3/1
  Embedded MATLAB Function2/1(dt1) -> Ialpha1/1, dt1/1

== system sensorless/SVPWM3/Subsystem ==
  to1 : Inport
  to2 : Inport  Port=2
  to3 : Inport  Port=3
  to4 : Inport  Port=4
  to5 : Inport  Port=5
  to6 : Inport  Port=6
  dt1 : Inport  Port=7
  dt2 : Inport  Port=8
  dt3 : Inport  Port=9
  tpwm : Inport  Port=10
  Current : Inport  Port=11
  Mux1 : Mux  Inputs=2
  Mux2 : Mux  Inputs=2
  Mux3 : Mux  Inputs=2
  Scope1 : Scope  NumInputPorts=3
  Scope2 : Scope  NumInputPorts=3
  Scope4 : Scope  NumInputPorts=3
  Subsystem1 : Subsystem
  Subsystem3 : Subsystem
  Subsystem4 : Subsystem
  frame Transformation for V1 abc-alpha_beta1 : MATLAB Function  TreatAsAtomicUnit=on
  frame Transformation for V1 abc-alpha_beta2 : MATLAB Function  TreatAsAtomicUnit=on
  frame Transformation for V1 abc-alpha_beta3 : MATLAB Function  TreatAsAtomicUnit=on
  di(alpha1) : Outport
  di(beta1) : Outport  Port=2
  di(alpha2) : Outport  Port=3
  di(beta2) : Outport  Port=4
  di(alpha0) : Outport  Port=5
  di(beta0) : Outport  Port=6
  wires:
  Subsystem3/6(Out6) -> frame Transformation for V1 abc-alpha_beta3/6(if1)
  Subsystem3/5(Out5) -> frame Transformation for V1 abc-alpha_beta3/5(ie)
  Subsystem3/1(Out1) -> frame Transformation for V1 abc-alpha_beta3/1(ia)
  Subsystem3/3(Out3) -> frame Transformation for V1 abc-alpha_beta3/3(ic)
  Subsystem3/2(Out2) -> frame Transformation for V1 abc-alpha_beta3/2(ib)
  Subsystem3/4(Out4) -> frame Transformation for V1 abc-alpha_beta3/4(id)
  to6/1 -> Subsystem3/2(t2)
  frame Transformation for V1 abc-alpha_beta1/2(I_beta_dV1) -> Mux3/2, di(beta1)/1
  frame Transformation for V1 abc-alpha_beta1/1(I_alpha_dV1) -> Mux3/1, di(alpha1)/1
  Current/1 -> Subsystem1/5(phase currents), Subsystem3/5(phase currents), Subsystem4/5(phase currents)
  dt1/1 -> Scope1/3, Subsystem4/4(dt1)
  tpwm/1 -> Subsystem3/3(tpwm), Subsystem1/3(tpwm), Subsystem4/3(tpwm)
  to2/1 -> Scope1/2, Subsystem4/2(t2)
  to1/1 -> Scope1/1, Subsystem4/1(t1)
  frame Transformation for V1 abc-alpha_beta3/2(I_beta_dV1) -> Mux2/2, di(beta0)/1
  frame Transformation for V1 abc-alpha_beta3/1(I_alpha_dV1) -> Mux2/1, di(alpha0)/1
  Subsystem1/5(Out5) -> frame Transformation for V1 abc-alpha_beta2/5(ie)
  Subsystem1/3(Out3) -> frame Transformation for V1 abc-alpha_beta2/3(ic)
  Subsystem1/1(Out1) -> frame Transformation for V1 abc-alpha_beta2/1(ia)
  Subsystem1/6(Out6) -> frame Transformation for V1 abc-alpha_beta2/6(if1)
  to5/1 -> Subsystem3/1(t1)
  to4/1 -> Subsystem1/2(t2)
  to3/1 -> Subsystem1/1(t1)
  Subsystem4/4(Out4) -> frame Transformation for V1 abc-alpha_beta1/4(id)
  Subsystem4/2(Out2) -> Scope2/2, frame Transformation for V1 abc-alpha_beta1/2(ib)
  Subsystem4/3(Out3) -> Scope2/3, frame Transformation for V1 abc-alpha_beta1/3(ic)
  Subsystem4/5(Out5) -> frame Transformation for V1 abc-alpha_beta1/5(ie)
  Subsystem4/1(Out1) -> Scope2/1, frame Transformation for V1 abc-alpha_beta1/1(ia)
  Subsystem4/6(Out6) -> frame Transformation for V1 abc-alpha_beta1/6(if1)
  frame Transformation for V1 abc-alpha_beta2/2(I_beta_dV1) -> Mux1/2, di(beta2)/1
  frame Transformation for V1 abc-alpha_beta2/1(I_alpha_dV1) -> Mux1/1, di(alpha2)/1
  Subsystem1/2(Out2) -> frame Transformation for V1 abc-alpha_beta2/2(ib)
  Subsystem1/4(Out4) -> frame Transformation for V1 abc-alpha_beta2/4(id)
  dt2/1 -> Subsystem1/4(dt1)
  dt3/1 -> Subsystem3/4(dt1)
  Mux3/1 -> Scope4/1
  Mux1/1 -> Scope4/2
  Mux2/1 -> Scope4/3

== system sensorless/SVPWM3/average ==
  In1 : Inport
  Delay5 : Delay  InitialCondition=0  SampleTime=1e-4
  Fcn1 : Fcn  Expr=5000*(u(1)-u(2))
  Mux2 : Mux  Inputs=2
  PID Controller2 : simulink/Continuous/PID Controller  Controller=I  Form=Parallel  TimeDomain=Continuous-time  SampleTime=-1  IntegratorMethod=Forward Euler  FilterMethod=Forward Euler  ControllerParametersSource=internal  P=1  I=1  D=0  UseFilter=on  N=100  TunerSelectOption=Transfer Function Based (PID Tuner App)  InitialConditionSource=internal  InitialConditionForIntegrator=0  InitialConditionForFilter=0  DifferentiatorICPrevScaledInput=0  ExternalReset=none  TrackingMode=off  Kt=1  LimitOutput=off  UpperSaturationLimit=inf  LowerSaturationLimit=-inf  LinearizeAsGain=on  AntiWindupMode=none  Kb=1  POutMin=[]  POutMax=[]  IOutMin=[]  IOutMax=[]  DOutMin=[]  DOutMax=[]  NOutMin=[]  NOutMax=[]  SumOutMin=[]  SumOutMax=[]  SaturationOutMin=[]  SaturationOutMax=[]  PParamMin=[]  PParamMax=[]  IParamMin=[]  IParamMax=[]  DParamMin=[]  DParamMax=[]  NParamMin=[]  NParamMax=[]  KbParamMin=[]  KbParamMax=[]  KtParamMin=[]  KtParamMax=[]  KbOutMin=[]  KbOutMax=[]  KtOutMin=[]  KtOutMax=[]  IntegratorOutMin=[]  IntegratorOutMax=[]  FilterOutMin=[]  FilterOutMax=[]  SumI1OutMin=[]  SumI1OutMax=[]  SumI2OutMin=[]  SumI2OutMax=[]  SumI3OutMin=[]  SumI3OutMax=[]  SumI4OutMin=[]  SumI4OutMax=[]  SumDOutMin=[]  SumDOutMax=[]  DifferentiatorOutMin=[]  DifferentiatorOutMax=[]  FilterDiffOutCoefMin=[]  FilterDiffOutCoefMax=[]  ReciprocalOutMin=[]  ReciprocalOutMax=[]  SumDenOutMin=[]  SumDenOutMax=[]  SumNumOutMin=[]  SumNumOutMax=[]  DivideOutMin=[]  DivideOutMax=[]  IntegratorContinuousStateAttributes=''  IntegratorStateMustResolveToSignalObject=off  IntegratorRTWStateStorageClass=Auto  FilterContinuousStateAttributes=''  FilterStateMustResolveToSignalObject=off  FilterRTWStateStorageClass=Auto  ParallelPVariant=Disabled  IdealPVariant=Disabled  IVariant=InternalParameters  DVariant=Disabled  IntegratorVariant=Continuous  SatVariant=Disabled  AWVariant=Passthrough  PCopyVariant=Disabled  TRVariant=Disabled  FdbkBlocksVariant=Forward  IdealPFdbkVariant=Disabled  SatFdbkVariant=Disabled  DerivativeFilterVariant=Disabled  NVariant=Disabled  NCopyVariant=Disabled_SignalSpec  FilterICVariant=Disabled  IntegratorICVariant=InternalICs  ExternalResetVariant=Disabled  TRSumVariant=Passthrough  SumFdbkVariant=Disabled  SumVariant=Passthrough_I
  PID Controller3 : simulink/Continuous/PID Controller  Controller=I  Form=Parallel  TimeDomain=Continuous-time  SampleTime=-1  IntegratorMethod=Forward Euler  FilterMethod=Forward Euler  ControllerParametersSource=internal  P=1  I=1  D=0  UseFilter=on  N=100  TunerSelectOption=Transfer Function Based (PID Tuner App)  InitialConditionSource=internal  InitialConditionForIntegrator=0  InitialConditionForFilter=0  DifferentiatorICPrevScaledInput=0  ExternalReset=none  TrackingMode=off  Kt=1  LimitOutput=off  UpperSaturationLimit=inf  LowerSaturationLimit=-inf  LinearizeAsGain=on  AntiWindupMode=none  Kb=1  POutMin=[]  POutMax=[]  IOutMin=[]  IOutMax=[]  DOutMin=[]  DOutMax=[]  NOutMin=[]  NOutMax=[]  SumOutMin=[]  SumOutMax=[]  SaturationOutMin=[]  SaturationOutMax=[]  PParamMin=[]  PParamMax=[]  IParamMin=[]  IParamMax=[]  DParamMin=[]  DParamMax=[]  NParamMin=[]  NParamMax=[]  KbParamMin=[]  KbParamMax=[]  KtParamMin=[]  KtParamMax=[]  KbOutMin=[]  KbOutMax=[]  KtOutMin=[]  KtOutMax=[]  IntegratorOutMin=[]  IntegratorOutMax=[]  FilterOutMin=[]  FilterOutMax=[]  SumI1OutMin=[]  SumI1OutMax=[]  SumI2OutMin=[]  SumI2OutMax=[]  SumI3OutMin=[]  SumI3OutMax=[]  SumI4OutMin=[]  SumI4OutMax=[]  SumDOutMin=[]  SumDOutMax=[]  DifferentiatorOutMin=[]  DifferentiatorOutMax=[]  FilterDiffOutCoefMin=[]  FilterDiffOutCoefMax=[]  ReciprocalOutMin=[]  ReciprocalOutMax=[]  SumDenOutMin=[]  SumDenOutMax=[]  SumNumOutMin=[]  SumNumOutMax=[]  DivideOutMin=[]  DivideOutMax=[]  IntegratorContinuousStateAttributes=''  IntegratorStateMustResolveToSignalObject=off  IntegratorRTWStateStorageClass=Auto  FilterContinuousStateAttributes=''  FilterStateMustResolveToSignalObject=off  FilterRTWStateStorageClass=Auto  ParallelPVariant=Disabled  IdealPVariant=Disabled  IVariant=InternalParameters  DVariant=Disabled  IntegratorVariant=Continuous  SatVariant=Disabled  AWVariant=Passthrough  PCopyVariant=Disabled  TRVariant=Disabled  FdbkBlocksVariant=Forward  IdealPFdbkVariant=Disabled  SatFdbkVariant=Disabled  DerivativeFilterVariant=Disabled  NVariant=Disabled  NCopyVariant=Disabled_SignalSpec  FilterICVariant=Disabled  IntegratorICVariant=InternalICs  ExternalResetVariant=Disabled  TRSumVariant=Passthrough  SumFdbkVariant=Disabled  SumVariant=Passthrough_I
  Out1 : Outport
  wires:
  Delay5/1 -> PID Controller3/1
  PID Controller3/1 -> Mux2/2
  PID Controller2/1 -> Mux2/1
  Mux2/1 -> Fcn1/1
  Fcn1/1 -> Out1/1
  In1/1 -> Delay5/1, PID Controller2/1

== system sensorless/dq-sixphasePMSM/dynamics ==
  note: Tem=p*(sqrt3*psi*iq+(Ld-Lq)*id*iq)
  load : Inport
  psi : Inport  Port=2
  iq : Inport  Port=3
  Ld : Inport  Port=4
  Lq : Inport  Port=5
  id : Inport  Port=6
  1/J : Gain  Gain=1/J  SaturateOnIntegerOverflow=on  OutDataTypeStr=Inherit: Same as input  ParamDataTypeStr=Inherit: Same as input
  30/pi : Gain  Gain=30/pi  SaturateOnIntegerOverflow=on  OutDataTypeStr=Inherit: Same as input  ParamDataTypeStr=Inherit: Same as input
  Constant : Constant  Value=pi
  Constant1 : Constant  Value=13*pi/9
  Fcn2 : Fcn  Expr=u(1)*(sqrt(3)*u(2)*u(3)+(u(4)-u(5))*u(6)*u(3))
  Integrator : Integrator  InitialConditionSource=external
  Integrator3 : Integrator
  Math Function : Math  Operator=mod  SaturateOnIntegerOverflow=on
  Mux1 : Mux  Inputs=6
  Sum3 : Sum  Inputs=|+-  SaturateOnIntegerOverflow=on
  "Theta Generator (-pi, pi)" : Subsystem
  p : Constant  Value=p
  pole : Gain  Gain=p  SaturateOnIntegerOverflow=on  OutDataTypeStr=Inherit: Same as input  ParamDataTypeStr=Inherit: Same as input
  u2 : Scope
  w : Outport
  n : Outport  Port=2
  Tem : Outport  Port=3
  tag scope: rp=global
  wires:
  p/1 -> Mux1/1
  Mux1/1 -> Fcn2/1
  Fcn2/1 -> Sum3/1, Tem/1
  Sum3/1 -> 1/J/1
  1/J/1 -> Integrator3/1
  Integrator3/1 -> 30/pi/1, pole/1
  psi/1 -> Mux1/2
  Ld/1 -> Mux1/4
  Lq/1 -> Mux1/5
  30/pi/1 -> n/1
  load/1 -> Sum3/2
  iq/1 -> Mux1/3
  id/1 -> Mux1/6
  pole/1 -> Integrator/1, w/1
  Integrator/1 -> Math Function/1
  Constant/1 -> Math Function/2, "Theta Generator (-pi, pi)"/1(pi)
  Math Function/1 -> "Theta Generator (-pi, pi)"/2(In)
  Constant1/1 -> Integrator/2
  "Theta Generator (-pi, pi)"/1(Out) -> [rp], u2/1

== system sensorless/dq-sixphasePMSM/motor ==
  ua : Inport
  ub : Inport  Port=2
  uc : Inport  Port=3
  ud : Inport  Port=4
  ue : Inport  Port=5
  uf : Inport  Port=6
  w : Inport  Port=7
  Integrator : Integrator
  Mux : Mux  Inputs=7
  Sum : Sum  Inputs=|++  SaturateOnIntegerOverflow=on
  initial angel : Step  Time=0  After=13*pi/9  SampleTime=0
  phase : Outport
  u : Outport  Port=2
  tag scope: phase=global
  wires:
  Sum/1 -> [phase], phase/1, Mux/7
  Integrator/1 -> Sum/1
  w/1 -> Integrator/1
  Mux/1 -> u/1
  ud/1 -> Mux/1
  ua/1 -> Mux/2
  ue/1 -> Mux/3
  ub/1 -> Mux/4
  uf/1 -> Mux/5
  uc/1 -> Mux/6
  initial angel/1 -> Sum/2

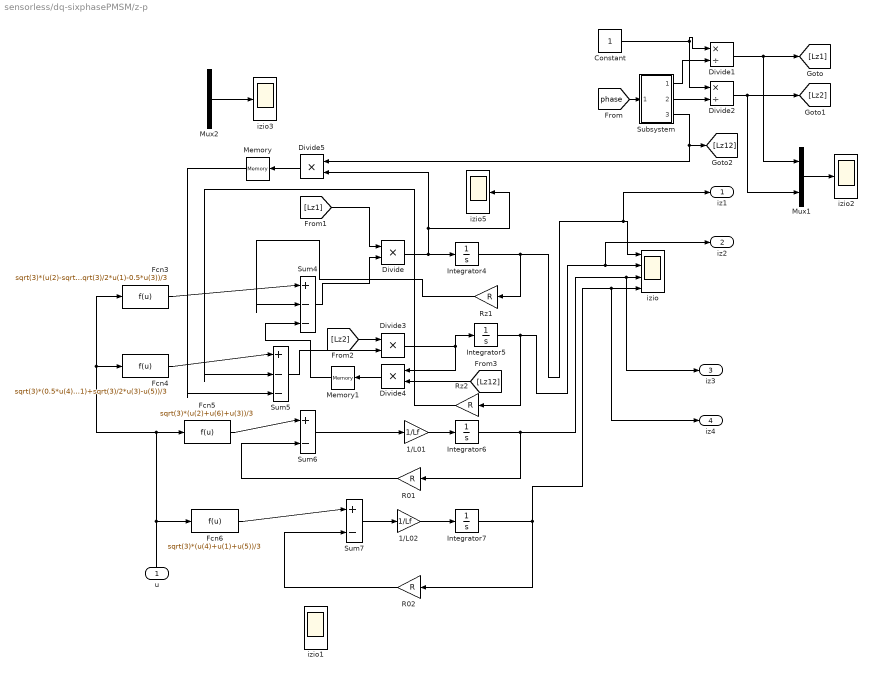
== system sensorless/dq-sixphasePMSM/z-p ==
  u : Inport
  1/L01 : Gain  Gain=1/Lf  SaturateOnIntegerOverflow=on  OutDataTypeStr=Inherit: Same as input  ParamDataTypeStr=Inherit: Same as input
  1/L02 : Gain  Gain=1/Lf  SaturateOnIntegerOverflow=on  OutDataTypeStr=Inherit: Same as input  ParamDataTypeStr=Inherit: Same as input
  Constant : Constant
  Divide{,3..5} (4 alike) : Product  Inputs=**
  Divide1 : Product  Inputs=*/
  Divide2 : Product  Inputs=*/
  Fcn3 : Fcn  Expr=sqrt(3)*(u(2)-sqrt(3)/2*u(4)-0.5*u(6)+sqrt(3)/2*u(1)-0.5*u(3))/3
  Fcn4 : Fcn  Expr=sqrt(3)*(0.5*u(4)-sqrt(3)/2*u(6)+0.5*u(1)+sqrt(3)/2*u(3)-u(5))/3
  Fcn5 : Fcn  Expr=sqrt(3)*(u(2)+u(6)+u(3))/3
  Fcn6 : Fcn  Expr=sqrt(3)*(u(4)+u(1)+u(5))/3
  Integrator{4..7} (4 alike) : Integrator
  Memory : Memory
  Memory1 : Memory
  Mux1 : Mux  Inputs=2
  Mux2 : Mux  Inputs=2
  R01 : Gain  Gain=R  SaturateOnIntegerOverflow=on  OutDataTypeStr=Inherit: Same as input  ParamDataTypeStr=Inherit: Same as input
  R02 : Gain  Gain=R  SaturateOnIntegerOverflow=on  OutDataTypeStr=Inherit: Same as input  ParamDataTypeStr=Inherit: Same as input
  Rz1 : Gain  Gain=R  SaturateOnIntegerOverflow=on  OutDataTypeStr=Inherit: Same as input  ParamDataTypeStr=Inherit: Same as input
  Rz2 : Gain  Gain=R  SaturateOnIntegerOverflow=on  OutDataTypeStr=Inherit: Same as input  ParamDataTypeStr=Inherit: Same as input
  Subsystem : Subsystem
  Sum4 : Sum  Inputs=|+--  SaturateOnIntegerOverflow=on
  Sum5 : Sum  Inputs=|+--  SaturateOnIntegerOverflow=on
  Sum6 : Sum  Inputs=|+-  SaturateOnIntegerOverflow=on
  Sum7 : Sum  Inputs=|+-  SaturateOnIntegerOverflow=on
  izio : Scope  NumInputPorts=4
  izio1 : Scope  NumInputPorts=4
  izio2 : Scope
  izio3 : Scope
  izio5 : Scope
  iz1 : Outport
  iz2 : Outport  Port=2
  iz3 : Outport  Port=3
  iz4 : Outport  Port=4
  wires:
  R02/1 -> Sum7/2
  R01/1 -> Sum6/2
  Rz2/1 -> Sum5/2
  Rz1/1 -> Sum4/2
  Integrator7/1 -> iz4/1, izio/4, R02/1
  1/L02/1 -> Integrator7/1
  Sum7/1 -> 1/L02/1
  Integrator6/1 -> iz3/1, izio/3, R01/1
  1/L01/1 -> Integrator6/1
  Sum6/1 -> 1/L01/1
  u/1 -> Fcn3/1, Fcn4/1, Fcn5/1, Fcn6/1
  [phase] -> Subsystem/1(Phase)
  Subsystem/1(Lz1) -> Divide1/2
  Divide1/1 -> Mux1/1, [Lz1]
  Constant/1 -> Divide1/1, Divide2/1
  Subsystem/2(Lz2) -> Divide2/2
  Divide2/1 -> Mux1/2, [Lz2]
  Mux1/1 -> izio2/1
  Sum4/1 -> Divide/2
  [Lz1] -> Divide/1
  Divide/1 -> izio5/1, Divide5/2, Integrator4/1
  Divide3/1 -> Integrator5/1, Divide4/1
  Sum5/1 -> Divide3/2
  [Lz2] -> Divide3/1
  Fcn5/1 -> Sum6/1
  Integrator5/1 -> Rz2/1, iz2/1, izio/2
  Integrator4/1 -> Rz1/1, iz1/1, izio/1
  Fcn4/1 -> Sum5/1
  Subsystem/3(Lz1z2) -> Divide5/1, [Lz12]
  Divide4/1 -> Memory1/1
  [Lz12] -> Divide4/2
  Divide5/1 -> Memory/1
  Memory1/1 -> Sum4/3
  Fcn6/1 -> Sum7/1
  Mux2/1 -> izio3/1
  Fcn3/1 -> Sum4/1
  Memory/1 -> Sum5/3

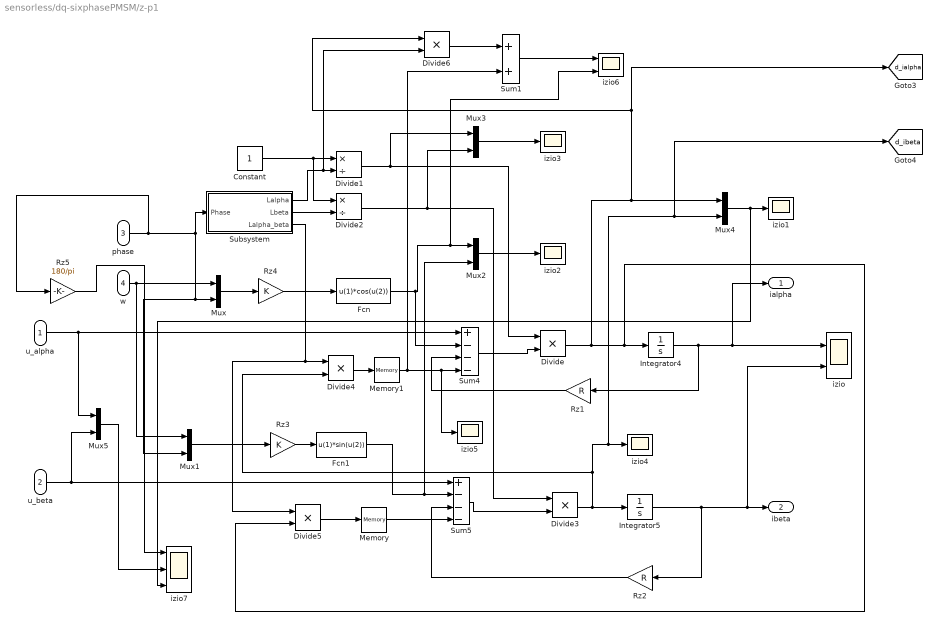
== system sensorless/dq-sixphasePMSM/z-p1 ==
  u_alpha : Inport
  u_beta : Inport  Port=2
  phase : Inport  Port=3
  w : Inport  Port=4
  Constant : Constant
  Divide{,3..6} (5 alike) : Product  Inputs=**
  Divide1 : Product  Inputs=*/
  Divide2 : Product  Inputs=*/
  Fcn : Fcn  Expr=u(1)*cos(u(2))
  Fcn1 : Fcn  Expr=u(1)*sin(u(2))
  Integrator4 : Integrator
  Integrator5 : Integrator
  Memory : Memory
  Memory1 : Memory
  Mux{,1..5} (6 alike) : Mux  Inputs=2
  Rz1 : Gain  Gain=R  SaturateOnIntegerOverflow=on  OutDataTypeStr=Inherit: Same as input  ParamDataTypeStr=Inherit: Same as input
  Rz2 : Gain  Gain=R  SaturateOnIntegerOverflow=on  OutDataTypeStr=Inherit: Same as input  ParamDataTypeStr=Inherit: Same as input
  Rz3 : Gain  Gain=K  SaturateOnIntegerOverflow=on  OutDataTypeStr=Inherit: Same as input  ParamDataTypeStr=Inherit: Same as input
  Rz4 : Gain  Gain=K  SaturateOnIntegerOverflow=on  OutDataTypeStr=Inherit: Same as input  ParamDataTypeStr=Inherit: Same as input
  Rz5 : Gain  Gain=180/pi  SaturateOnIntegerOverflow=on  OutDataTypeStr=Inherit: Same as input  ParamDataTypeStr=Inherit: Same as input
  Subsystem : Subsystem
  Sum1 : Sum  SaturateOnIntegerOverflow=on
  Sum4 : Sum  Inputs=+---  SaturateOnIntegerOverflow=on
  Sum5 : Sum  Inputs=+---  SaturateOnIntegerOverflow=on
  izio : Scope  NumInputPorts=2
  izio{1..5} (5 alike) : Scope
  izio6 : Scope  NumInputPorts=2
  izio7 : Scope  NumInputPorts=3
  ialpha : Outport
  ibeta : Outport  Port=2
  tag scope: d_ialpha=global, d_ibeta=global
  wires:
  phase/1 -> Rz5/1, Subsystem/1(Phase), Mux1/2, Mux/2
  Subsystem/1(Lalpha) -> Divide6/2, Divide1/2
  Constant/1 -> Divide1/1, Divide2/1
  Subsystem/2(Lbeta) -> Divide2/2
  Sum4/1 -> Divide/2
  Divide/1 -> Divide6/1, [d_ialpha], Mux4/1, Divide5/2, Integrator4/1
  Divide3/1 -> [d_ibeta], Mux4/2, izio4/1, Divide4/2, Integrator5/1
  Sum5/1 -> Divide3/2
  Integrator4/1 -> Rz1/1, ialpha/1, izio/1
  Rz1/1 -> Sum4/3
  Rz2/1 -> Sum5/3
  u_alpha/1 -> Mux5/1, Sum4/1
  u_beta/1 -> Mux5/2, Sum5/1
  Divide1/1 -> Mux3/1, Divide/1
  Divide2/1 -> Mux3/2, Divide3/1
  w/1 -> Mux/1, Mux1/1
  Mux/1 -> Rz4/1
  Fcn/1 -> Sum4/2, izio6/2, Mux2/1
  Fcn1/1 -> Mux2/2, Sum5/2
  Mux1/1 -> Rz3/1
  Divide4/1 -> Memory1/1
  Subsystem/3(Lalpha_beta) -> Divide4/1, Divide5/1
  Integrator5/1 -> Rz2/1, izio/2, ibeta/1
  Divide5/1 -> Memory/1
  Mux2/1 -> izio2/1
  Mux3/1 -> izio3/1
  Mux4/1 -> izio7/3, izio1/1
  Memory/1 -> Sum5/4
  Memory1/1 -> izio5/1, Sum4/4, Sum1/2
  Rz3/1 -> Fcn1/1
  Rz4/1 -> Fcn/1
  Divide6/1 -> Sum1/1
  Sum1/1 -> izio6/1
  Rz5/1 -> izio7/1
  Mux5/1 -> izio7/2
